simulink model "Seilwinde"  (R2020a)
settings: Solver=FixedStepAuto  StartTime=0.0  StopTime=tend_sim  FixedStep=stepsize  RelTol=1e-3
undefined symbols (not defined in the file): d_visc, i_Getriebe, I_max_eff, i_Seilwinde, J_Lastwinde, K_m, K_p, K_pi2, K_s, k_stat, K_v, R, R_Trommel, stepsize, T_el, T_i_control, T_n, T_ni2, T_tot, T_v_control, T_x_control, U_z
settings Model: Creator=DELL  LastModifiedBy=rausc
settings DataIOCC: ReturnWorkspaceOutputs=off
settings DebuggingCC: ArithmeticOperatorsInVariantConditions=warning
settings SFSimCC: CustomCodeUndefinedFunction=UseInterfaceOnly

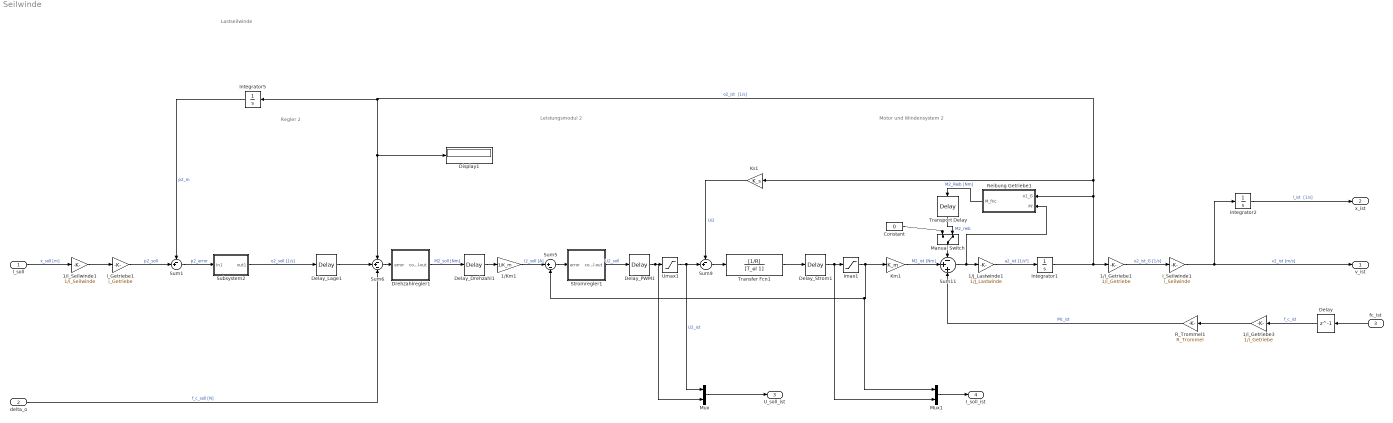
== system Seilwinde ==
  note: Regler 2
  note: Leistungsmodul 2
  note: Lastseilwinde
  note: Motor und Windensystem 2
  l_soll : Inport
  "delta_o " : Inport  Port=2
  fc_ist : Inport  Port=3
  1/J_Lastwinde1 : Gain  Gain=1/J_Lastwinde
  1/Km1 : Gain  Gain=1/K_m
  1/i_Getriebe1 : Gain  Gain=1/i_Getriebe
  1/i_Getriebe3 : Gain  Gain=1/i_Getriebe
  1/i_Seilwinde1 : Gain  Gain=1/i_Seilwinde
  Constant : Constant  Value=0
  Delay : Delay  DelayLength=1
  Delay_Drehzahl1 : TransportDelay  DelayTime=T_v_control
  Delay_Lage1 : TransportDelay  DelayTime=T_x_control
  Delay_PWM1 : TransportDelay  DelayTime=T_tot
  Delay_Strom1 : TransportDelay  DelayTime=T_i_control
  Display1 : Display
  Drehzahlregler1 : Subsystem  mask{gain=K_p, time_constant=T_n}
      mask prompts: time_constant "Time Constant"
      mask Display: disp('PI Controller');
  Imax1 : Saturate  UpperLimit=I_max_eff  LowerLimit=-I_max_eff
  Integrator1 : Integrator
  Integrator2 : Integrator
  Integrator5 : Integrator
  Km1 : Gain  Gain=K_m
  Ks1 : Gain  Gain=K_s
  Manual Switch : ManualSwitch  CurrentSetting=0
  Mux : Mux  Inputs=2
  Mux1 : Mux  Inputs=2
  R_Trommel1 : Gain  Gain=R_Trommel
  Reibung Getriebe1 : Subsystem
  Stromregler1 : Subsystem  mask{gain=K_pi2, time_constant=T_ni2}
      mask prompts: time_constant "Time Constant"
      mask Display: disp('PI Controller');
  Subsystem2 : Subsystem  mask{gain=K_v}
      mask Display: disp('P Controller')
  Sum1 : Sum  Inputs=-+|
  Sum11 : Sum  Inputs=-++
  Sum5 : Sum  Inputs=|+-
  Sum6 : Sum  Inputs=-+-
  Sum9 : Sum  Inputs=-+|
  Transfer Fcn1 : TransferFcn  Numerator=[1/R]  Denominator=[T_el 1]  ContinuousStateAttributes='current'
  Transport Delay : TransportDelay  DelayTime=stepsize
  Umax1 : Saturate  UpperLimit=U_z  LowerLimit=-U_z
  i_Getriebe1 : Gain  Gain=i_Getriebe
  i_Seilwinde1 : Gain  Gain=i_Seilwinde
  "v_ist " : Outport
  x_ist : Outport  Port=2
  U_soll_ist : Outport  Port=3
  I_soll_ist : Outport  Port=4
  wires:
  Sum1/1 -> Subsystem2/1(In1)  "p2_error"
  Km1/1 -> Sum11/2  "M2_ist [Nm]"
  Delay_Drehzahl1/1 -> 1/Km1/1
  Transport Delay/1 -> Manual Switch/2  "M2_reib"
  1/i_Getriebe3/1 -> R_Trommel1/1
  i_Getriebe1/1 -> Sum1/2  "p2_soll"
  Integrator5/1 -> Sum1/1  "p2_m"
  Sum5/1 -> Stromregler1/1(error)
  1/i_Seilwinde1/1 -> i_Getriebe1/1
  Ks1/1 -> Sum9/1  "Ui2"
  Subsystem2/1("out1 ") -> Delay_Lage1/1  "o2_soll [1/s]"
  l_soll/1 -> 1/i_Seilwinde1/1  "x_soll [m]"
  Drehzahlregler1/1(control-out) -> Delay_Drehzahl1/1  "M2_soll [Nm]"
  Delay_PWM1/1 -> Mux/2, Umax1/1
  Sum6/1 -> Drehzahlregler1/1(error)
  Umax1/1 -> Mux/1, Sum9/2  "U2_ist"
  1/i_Getriebe1/1 -> i_Seilwinde1/1  "o2_ist_G [1/s]"
  1/Km1/1 -> Sum5/1  "I2_soll [A]"
  Stromregler1/1(control-out) -> Delay_PWM1/1  "U2_soll"
  Integrator1/1 -> Reibung Getriebe1/1(o1_G), Sum6/1, Display1/1, Integrator5/1, Ks1/1, 1/i_Getriebe1/1  "o2_ist  [1/s]"
  1/J_Lastwinde1/1 -> Integrator1/1  "a2_ist [1/s²]"
  Sum11/1 -> Reibung Getriebe1/2(M'), 1/J_Lastwinde1/1
  Reibung Getriebe1/1(M_fric) -> Transport Delay/1  "M2_Reib [Nm]"
  i_Seilwinde1/1 -> Integrator2/1, "v_ist "/1  "v2_ist [m/s]"
  R_Trommel1/1 -> Sum11/3  "Mc_ist"
  Sum9/1 -> Transfer Fcn1/1
  Transfer Fcn1/1 -> Delay_Strom1/1
  fc_ist/1 -> Delay/1
  Delay/1 -> 1/i_Getriebe3/1  "f_c_ist"
  Delay_Lage1/1 -> Sum6/2
  Integrator2/1 -> x_ist/1  "l_ist  [1/s]"
  "delta_o "/1 -> Sum6/3  "f_c_soll [N]"
  Constant/1 -> Manual Switch/1
  Manual Switch/1 -> Sum11/1
  Imax1/1 -> Mux1/1, Sum5/2, Km1/1
  Delay_Strom1/1 -> Mux1/2, Imax1/1
  Mux1/1 -> I_soll_ist/1
  Mux/1 -> U_soll_ist/1

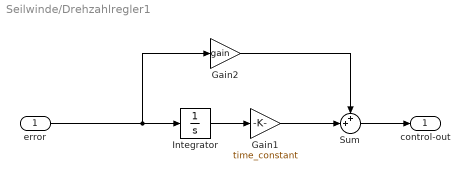
== system Seilwinde/Drehzahlregler1 ==
  error : Inport
  Gain1 : Gain  Gain=time_constant
  Gain2 : Gain  Gain=gain
  Integrator : Integrator
  Sum : Sum  Inputs=++|
  control-out : Outport
  wires:
  Sum/1 -> control-out/1
  Gain2/1 -> Sum/1
  error/1 -> Integrator/1, Gain2/1
  Integrator/1 -> Gain1/1
  Gain1/1 -> Sum/2

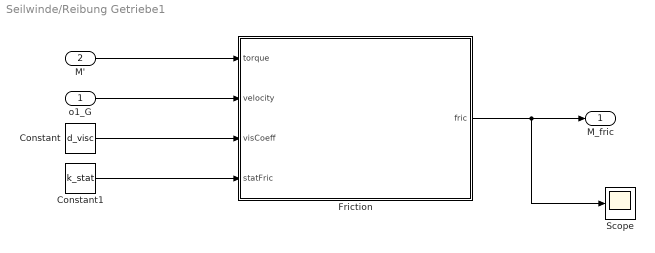
== system Seilwinde/Reibung Getriebe1 ==
  o1_G : Inport
  M' : Inport  Port=2
  Constant : Constant  Value=d_visc
  Constant1 : Constant  Value=k_stat
  Friction : MATLAB Function  TreatAsAtomicUnit=on
  Scope : Scope
  M_fric : Outport  VectorParamsAs1DForOutWhenUnconnected=off
  wires:
  Constant/1 -> Friction/3(visCoeff)
  o1_G/1 -> Friction/2(velocity)
  M'/1 -> Friction/1(torque)
  Friction/1(fric) -> Scope/1, M_fric/1
  Constant1/1 -> Friction/4(statFric)

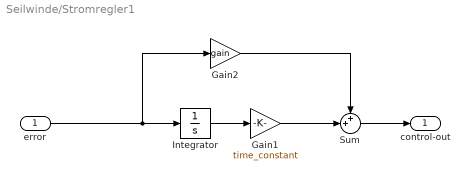
== system Seilwinde/Stromregler1 ==
  error : Inport
  Gain1 : Gain  Gain=time_constant
  Gain2 : Gain  Gain=gain
  Integrator : Integrator
  Sum : Sum  Inputs=++|
  control-out : Outport
  wires:
  Sum/1 -> control-out/1
  Gain2/1 -> Sum/1
  error/1 -> Integrator/1, Gain2/1
  Integrator/1 -> Gain1/1
  Gain1/1 -> Sum/2

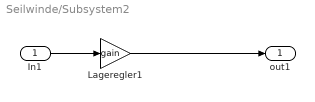
== system Seilwinde/Subsystem2 ==
  In1 : Inport
  Lageregler1 : Gain  Gain=gain
  "out1 " : Outport
  wires:
  In1/1 -> Lageregler1/1
  Lageregler1/1 -> "out1 "/1

== matlab function Seilwinde/Reibung Getriebe1/Friction ==
  data: torque input; velocity input; visCoeff input; statFric input; fric output
%% Viskose Reibung/Stokesreibung
function fric   = fcn(torque, velocity,visCoeff,statFric)

   if abs(velocity) < 0.01
    if torque > statFric
      fric = statFric;
    elseif torque < -statFric
      fric = -statFric;
    else
      fric = torque;
    end   
  else 
    fric = statFric*sign(velocity) + visCoeff*velocity*sign(velocity);   
   end 
  
end
%% Stribeck-Effekt
% function fric   = fcn(torque, velocity,visCoeff,statFric)
% fc = 0.8*statFric; 
%   if abs(velocity) < 0.00001
%     if torque > statFric
%       fric = statFric;
%     elseif torque < -statFric
%       fric = -statFric;
%     else %-statFric < torque_R && torque_R < statFric
%       fric = torque;
%     end
%     
%   else %if abs(velocity) < 0.001 && abs(velocity) > 0
%      fric = (fc + (statFric-fc)*exp(-abs(velocity/0.001))) ...
%        *sign(velocity) + visCoeff*velocity;
% %   else
% %   fric = statFric*sign(velocity) + visCoeff*velocity;
%   end
% end
